simulink model "AVION_LONGITUDINAL"  (Simulink 8.2)
settings: Solver=ode45  StartTime=0.0  StopTime=100  RelTol=1e-8
values from neighbouring files (symbols this model uses):
  ACinertia_yy = 8000.0    (= 8000)    [iniAVION_LONGITUDINAL.m]
  ACmass = 90000.0    (= 90000)    [iniAVION_LONGITUDINAL.m]
  ae = Ue(2)    [iniAVION_LONGITUDINAL.m]
  cbar = 5.0    (= 5)    [iniAVION_LONGITUDINAL.m]
  CD0 = 0.018    [iniAVION_LONGITUDINAL.m]
  CD1 = 0.009    [iniAVION_LONGITUDINAL.m]
  CD2 = 0.040    (= 0.04)    [iniAVION_LONGITUDINAL.m]
  CL0 = 0.20    (= 0.2)    [iniAVION_LONGITUDINAL.m]
  CLalfa = 0.20    (= 0.2)    [iniAVION_LONGITUDINAL.m]
  CM0 = 0.050    (= 0.05)    [iniAVION_LONGITUDINAL.m]
  CMalfa = -0.001    [iniAVION_LONGITUDINAL.m]
  CMdelta = -0.016    [iniAVION_LONGITUDINAL.m]
  CMq = -0.300    (= -0.3)    [iniAVION_LONGITUDINAL.m]
  d2r_cst = pi/180.0    (= 0.0174532925199)    [iniAVION_LONGITUDINAL.m]
  deltae = Ue(1)    [iniAVION_LONGITUDINAL.m]
  etat_ini = etat_equil    [iniAVION_LONGITUDINAL.m]
  FT80 = thrust_max    (= 108000)    [iniAVION_LONGITUDINAL.m]
  FT_V = -200.0    (= -200)    [iniAVION_LONGITUDINAL.m]
  g_cst = 9.78    [iniAVION_LONGITUDINAL.m]
  pos_ini = [h_ini, pN_ini]    [iniAVION_LONGITUDINAL.m]
  r2d_cst = 1.0/d2r_cst    (= 57.2957795131)    [iniAVION_LONGITUDINAL.m]
  rho = 1.225    [iniAVION_LONGITUDINAL.m]
  Sref = 200.0    (= 200)    [iniAVION_LONGITUDINAL.m]
  xt = -0.3    [iniAVION_LONGITUDINAL.m]
undefined symbols (not defined in the file or in its folder): A, B, C, D, Ye
settings Model: Creator=delafontaine  LastModifiedBy=Ouss
settings DataIOCC: SignalLoggingName=sigsOut
settings OptimizationCC: BooleanDataType=off
settings DebuggingCC: SaveWithParameterizedLinksMsg=none  SignalResolutionControl=TryResolveAllWithWarning  SolverPrmCheckMsg=none  MultiTaskDSMMsg=warning  MultiTaskCondExecSysMsg=none  FcnCallInpInsideContextMsg=EnableAllAsWarning  FrameProcessingCompatibilityMsg=error
settings HardwareCC: TargetUnknown=on
settings GRTTargetCC: CodeReplacementLibrary=None  CPPClassGenCompliant=on

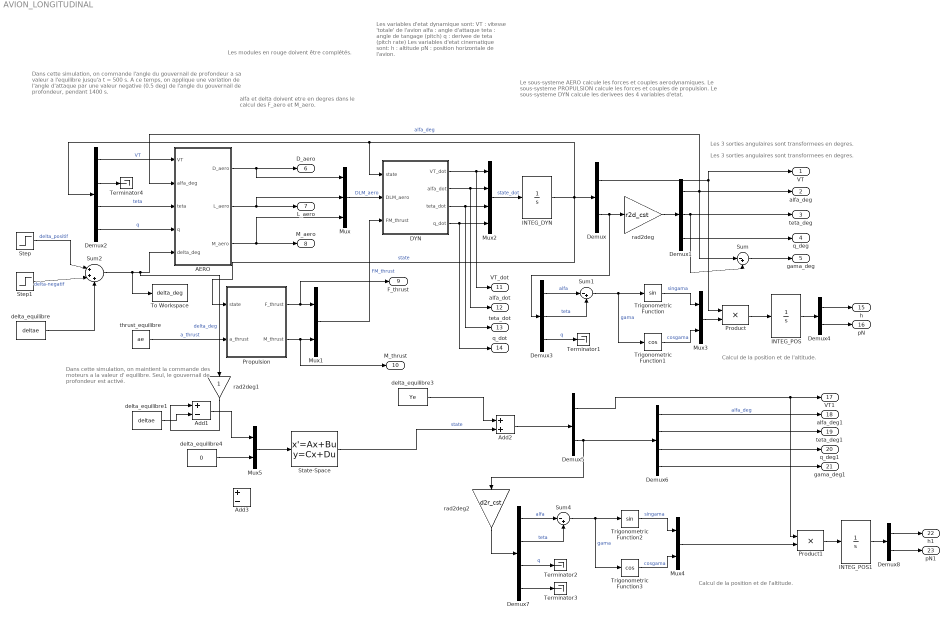
== system AVION_LONGITUDINAL ==
  note: Dans cette simulation, on commande l'angle du gouvernail
      | de profondeur a sa valeur a l'equilibre jusqu'a t = 500 s. A ce
      | temps, on applique une variation de l'angle d'attaque
      | par une valeur negative (0.5 deg) de l'angle du gouvernail
      | de profondeur, pendant 1400 s.
  note: alfa et delta doivent etre en degres
      | dans le calcul des F_aero et M_aero.
  note: Les variables d'etat dynamique sont:
      |
      | VT   : vitesse 'totale' de l'avion
      | alfa : angle d'attaque
      | teta : angle de tangage (pitch)
      | q    : derivee de teta (pitch rate)
      |
      | Les variables d'etat cinematique sont:
      |
      | h    : altitude
      | pN   : position horizontale de l'avion.
  note: Les 3 sorties angulaires sont transformees en degres.
  note: Calcul de la position et de l'altitude.
  note: Le sous-systeme AERO calcule les forces et couples
      | aerodynamiques. Le sous-systeme PROPULSION calcule
      | les forces et couples de propulsion. Le sous-systeme
      | DYN calcule les derivees des 4 variables d'etat.
  note: Dans cette simulation, on maintient la
      | commande des moteurs a la valeur d' equilibre.
      | Seul, le gouvernail de profondeur est activé.
  note: Les modules en rouge doivent être complétés.
  note: Les 3 sorties angulaires sont transformees en degres.
  note: Calcul de la position et de l'altitude.
  AERO : Subsystem
  Add1 : Sum  Inputs=+-
  Add2 : Sum
  Add3 : Sum  Inputs=+-
  DYN : Subsystem
  Demux : Demux  Outputs=[1,3]
  Demux1 : Demux  Outputs=3
  Demux2 : Demux
  Demux3 : Demux  Outputs=3
  Demux4 : Demux  Outputs=2
  Demux5 : Demux  Outputs=[1,4]
  Demux6 : Demux
  Demux7 : Demux
  Demux8 : Demux  Outputs=2
  INTEG_DYN : Integrator  InitialCondition=etat_ini
  INTEG_POS : Integrator  InitialCondition=pos_ini
  INTEG_POS1 : Integrator  InitialCondition=pos_ini
  Mux : Mux  Inputs=3
  Mux{1,3..5} (4 alike) : Mux  Inputs=2
  Mux2 : Mux
  Product : Product  Inputs=**  SaturateOnIntegerOverflow=on  InputSameDT=on  OutDataTypeStr=Inherit: Same as first input
  Product1 : Product  Inputs=**  SaturateOnIntegerOverflow=on  InputSameDT=on  OutDataTypeStr=Inherit: Same as first input
  Propulsion : Subsystem
  State-Space : StateSpace  A=A  B=B  C=C  D=D  X0=0  ContinuousStateAttributes='avionnn'
  Step : Step  Time=1900  After=0.5  SampleTime=0
  Step1 : Step  Time=500  After=-0.5  SampleTime=0
  Sum : Sum  Inputs=|-+  SaturateOnIntegerOverflow=on  InputSameDT=on  OutDataTypeStr=Inherit: Same as first input
  Sum1 : Sum  Inputs=|-+  SaturateOnIntegerOverflow=on  InputSameDT=on  OutDataTypeStr=Inherit: Same as first input
  Sum2 : Sum  Inputs=|+++  SaturateOnIntegerOverflow=on  InputSameDT=on  OutDataTypeStr=Inherit: Same as first input
  Sum4 : Sum  Inputs=|-+  SaturateOnIntegerOverflow=on  InputSameDT=on  OutDataTypeStr=Inherit: Same as first input
  Terminator{1..4} (4 alike) : Terminator
  To Workspace : ToWorkspace  VariableName=delta_deg  SampleTime=-1
  Trigonometric Function : Trigonometry
  Trigonometric Function1 : Trigonometry  Operator=cos
  Trigonometric Function2 : Trigonometry
  Trigonometric Function3 : Trigonometry  Operator=cos
  delta_equilibre : Constant  Value=deltae
  delta_equilibre1 : Constant  Value=deltae
  delta_equilibre3 : Constant  Value=Ye
  delta_equilibre4 : Constant  Value=0
  rad2deg : Gain  Gain=r2d_cst  SaturateOnIntegerOverflow=on  OutDataTypeStr=Inherit: Same as input  ParamDataTypeStr=Inherit: Same as input
  rad2deg1 : Gain  SaturateOnIntegerOverflow=on  OutDataTypeStr=Inherit: Same as input  ParamDataTypeStr=Inherit: Same as input
  rad2deg2 : Gain  Gain=d2r_cst  SaturateOnIntegerOverflow=on  OutDataTypeStr=Inherit: Same as input  ParamDataTypeStr=Inherit: Same as input
  thrust_equilibre : Constant  Value=ae
  VT : Outport
  alfa_deg : Outport  Port=2
  teta_deg : Outport  Port=3
  q_deg : Outport  Port=4
  gama_deg : Outport  Port=5
  D_aero : Outport  Port=6
  L_aero : Outport  Port=7
  M_aero : Outport  Port=8
  F_thrust : Outport  Port=9
  M_thrust : Outport  Port=10
  VT_dot : Outport  Port=11
  alfa_dot : Outport  Port=12
  teta_dot : Outport  Port=13
  q_dot : Outport  Port=14
  h : Outport  Port=15
  pN : Outport  Port=16
  VT1 : Outport  Port=17
  alfa_deg1 : Outport  Port=18
  teta_deg1 : Outport  Port=19
  q_deg1 : Outport  Port=20
  gama_deg1 : Outport  Port=21
  h1 : Outport  Port=22
  pN1 : Outport  Port=23
  wires:
  AERO/1(D_aero) -> D_aero/1, Mux/1
  AERO/2(L_aero) -> L_aero/1, Mux/2
  AERO/3(M_aero) -> M_aero/1, Mux/3
  Mux/1 -> DYN/2(DLM_aero)  "DLM_aero"
  Propulsion/1(F_thrust) -> Mux1/1, F_thrust/1
  Propulsion/2(M_thrust) -> Mux1/2, M_thrust/1
  Mux1/1 -> DYN/3(FM_thrust)  "FM_thrust"
  thrust_equilibre/1 -> Propulsion/2(a_thrust)  "a_thrust"
  DYN/1(VT_dot) -> Mux2/1, VT_dot/1
  DYN/2(alfa_dot) -> Mux2/2, alfa_dot/1
  DYN/3(teta_dot) -> Mux2/3, teta_dot/1
  DYN/4(q_dot) -> Mux2/4, q_dot/1
  Mux2/1 -> INTEG_DYN/1  "state_dot"
  INTEG_DYN/1 -> Demux/1, Demux2/1, DYN/1(state), Propulsion/1(state)  "state"
  Demux/2 -> rad2deg/1, Demux3/1
  Demux/1 -> Product/1, VT/1
  rad2deg/1 -> Demux1/1
  Demux1/1 -> AERO/2(alfa_deg), alfa_deg/1, Sum/1  "alfa_deg"
  Demux1/2 -> teta_deg/1, Sum/2
  Demux1/3 -> q_deg/1
  Sum/1 -> gama_deg/1
  Demux2/1 -> AERO/1(VT)  "VT"
  Demux2/3 -> AERO/3(teta)  "teta"
  Demux2/4 -> AERO/4(q)  "q"
  Sum1/1 -> Trigonometric Function/1, Trigonometric Function1/1  "gama"
  Trigonometric Function/1 -> Mux3/1  "singama"
  Trigonometric Function1/1 -> Mux3/2  "cosgama"
  INTEG_POS/1 -> Demux4/1
  Demux4/1 -> h/1
  Demux4/2 -> pN/1
  Demux3/3 -> Terminator1/1  "q"
  Demux3/1 -> Sum1/1  "alfa"
  Demux3/2 -> Sum1/2  "teta"
  delta_equilibre/1 -> Sum2/3
  Sum2/1 -> rad2deg1/1, AERO/5(delta_deg), To Workspace/1  "delta_deg"
  Step/1 -> Sum2/1  "delta_positif"
  Step1/1 -> Sum2/2  "delta-negatif"
  Mux3/1 -> Product/2
  Product/1 -> INTEG_POS/1
  Sum4/1 -> Trigonometric Function3/1, Trigonometric Function2/1  "gama"
  Trigonometric Function2/1 -> Mux4/1  "singama"
  Trigonometric Function3/1 -> Mux4/2  "cosgama"
  INTEG_POS1/1 -> Demux8/1
  Demux8/1 -> h1/1
  Demux8/2 -> pN1/1
  Demux7/3 -> Terminator2/1  "q"
  Demux7/1 -> Sum4/1  "alfa"
  Demux7/2 -> Sum4/2  "teta"
  Demux7/4 -> Terminator3/1
  Mux5/1 -> State-Space/1
  delta_equilibre1/1 -> Add1/2
  Add1/1 -> Mux5/1
  Demux6/1 -> alfa_deg1/1  "alfa_deg"
  Demux5/1 -> Product1/1, VT1/1
  Demux6/2 -> teta_deg1/1
  Demux6/3 -> q_deg1/1
  Demux6/4 -> gama_deg1/1
  Product1/1 -> INTEG_POS1/1
  rad2deg1/1 -> Add1/1
  Mux4/1 -> Product1/2
  rad2deg2/1 -> Demux7/1
  Add2/1 -> Demux5/1
  State-Space/1 -> Add2/2  "state"
  delta_equilibre3/1 -> Add2/1
  delta_equilibre4/1 -> Mux5/2
  Demux5/2 -> Demux6/1, rad2deg2/1
  Demux2/2 -> Terminator4/1

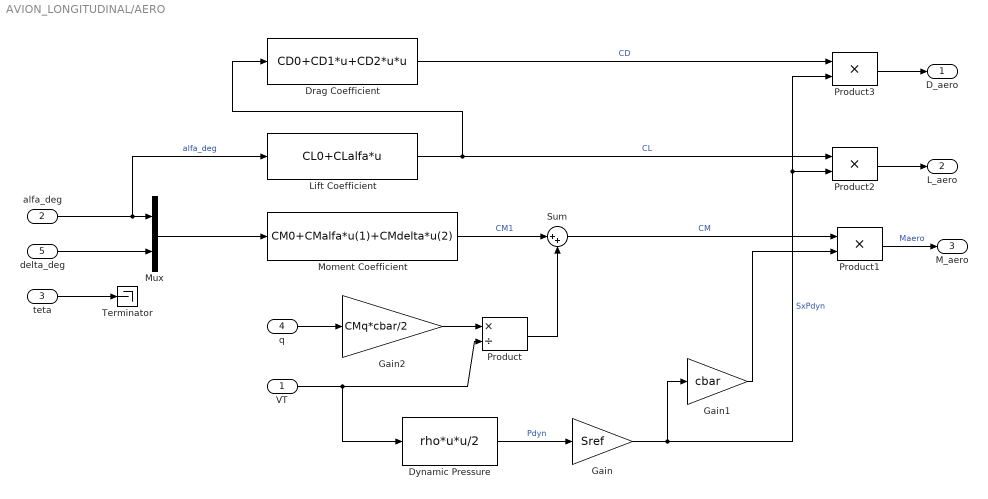
== system AVION_LONGITUDINAL/AERO ==
  VT : Inport
  alfa_deg : Inport  Port=2
  teta : Inport  Port=3
  q : Inport  Port=4
  delta_deg : Inport  Port=5
  Drag Coefficient : Fcn  Expr=CD0+CD1*u+CD2*u*u
  Dynamic Pressure : Fcn  Expr=rho*u*u/2
  Gain : Gain  Gain=Sref  SaturateOnIntegerOverflow=on  OutDataTypeStr=Inherit: Same as input  ParamDataTypeStr=Inherit: Same as input
  Gain1 : Gain  Gain=cbar  SaturateOnIntegerOverflow=on  OutDataTypeStr=Inherit: Same as input  ParamDataTypeStr=Inherit: Same as input
  Gain2 : Gain  Gain=CMq*cbar/2  SaturateOnIntegerOverflow=on  OutDataTypeStr=Inherit: Same as input  ParamDataTypeStr=Inherit: Same as input
  Lift Coefficient : Fcn  Expr=CL0+CLalfa*u
  Moment Coefficient : Fcn  Expr=CM0+CMalfa*u(1)+CMdelta*u(2)
  Mux : Mux  Inputs=2
  Product : Product  Inputs=*/  SaturateOnIntegerOverflow=on  InputSameDT=on  OutDataTypeStr=Inherit: Same as first input
  Product1 : Product  Inputs=**  SaturateOnIntegerOverflow=on  InputSameDT=on  OutDataTypeStr=Inherit: Same as first input
  Product2 : Product  Inputs=**  SaturateOnIntegerOverflow=on  InputSameDT=on  OutDataTypeStr=Inherit: Same as first input
  Product3 : Product  Inputs=**  SaturateOnIntegerOverflow=on  InputSameDT=on  OutDataTypeStr=Inherit: Same as first input
  Sum : Sum  Inputs=|++  SaturateOnIntegerOverflow=on  InputSameDT=on  OutDataTypeStr=Inherit: Same as first input
  Terminator : Terminator
  D_aero : Outport
  L_aero : Outport  Port=2
  M_aero : Outport  Port=3
  wires:
  Dynamic Pressure/1 -> Gain/1  "Pdyn"
  q/1 -> Gain2/1
  Gain2/1 -> Product/1
  VT/1 -> Product/2, Dynamic Pressure/1
  Product/1 -> Sum/2
  Moment Coefficient/1 -> Sum/1  "CM1"
  Sum/1 -> Product1/1  "CM"
  alfa_deg/1 -> Lift Coefficient/1, Mux/1  "alfa_deg"
  delta_deg/1 -> Mux/2
  Mux/1 -> Moment Coefficient/1
  Gain1/1 -> Product1/2
  Product1/1 -> M_aero/1  "Maero"
  Lift Coefficient/1 -> Drag Coefficient/1, Product2/1  "CL"
  Drag Coefficient/1 -> Product3/1  "CD"
  Product3/1 -> D_aero/1
  Product2/1 -> L_aero/1
  teta/1 -> Terminator/1
  Gain/1 -> Product2/2, Product3/2, Gain1/1  "SxPdyn"

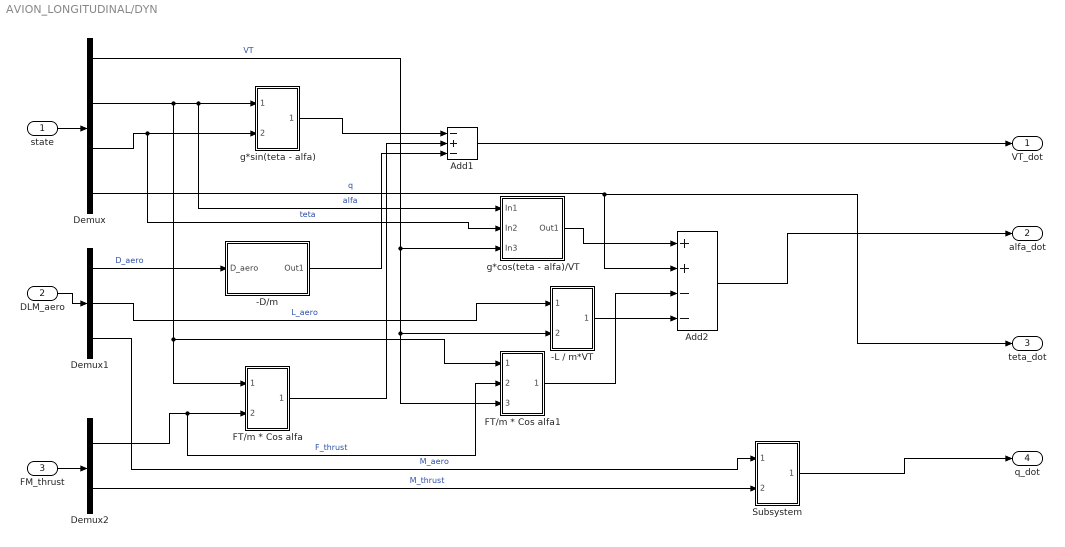
== system AVION_LONGITUDINAL/DYN ==
  state : Inport
  DLM_aero : Inport  Port=2
  FM_thrust : Inport  Port=3
  -D/m : Subsystem
  -L / m*VT : Subsystem
  Add1 : Sum  Inputs=-+-
  Add2 : Sum  Inputs=++--
  Demux : Demux
  Demux1 : Demux  Outputs=3
  Demux2 : Demux  Outputs=2
  FT/m * Cos alfa : Subsystem
  FT/m * Cos alfa1 : Subsystem
  Subsystem : Subsystem
  g*cos(teta - alfa)/VT : Subsystem
  g*sin(teta - alfa) : Subsystem
  VT_dot : Outport
  alfa_dot : Outport  Port=2
  teta_dot : Outport  Port=3
  q_dot : Outport  Port=4
  wires:
  state/1 -> Demux/1
  Demux/1 -> -L / m*VT/2(In2), FT/m * Cos alfa1/3(In3), g*cos(teta - alfa)/VT/3(In3)  "VT"
  DLM_aero/1 -> Demux1/1
  FM_thrust/1 -> Demux2/1
  Demux/2 -> FT/m * Cos alfa1/1(In1), FT/m * Cos alfa/1(In1), g*cos(teta - alfa)/VT/1(In1), g*sin(teta - alfa)/1(In1)  "alfa"
  Demux/4 -> teta_dot/1, Add2/2  "q"
  Demux1/2 -> -L / m*VT/1(In1)  "L_aero"
  Add1/1 -> VT_dot/1
  Demux2/1 -> FT/m * Cos alfa1/2(In2), FT/m * Cos alfa/2(In2)  "F_thrust"
  FT/m * Cos alfa/1(Out1) -> Add1/2
  Demux1/1 -> -D/m/1("D_aero ")  "D_aero"
  -D/m/1(Out1) -> Add1/3
  Demux/3 -> g*cos(teta - alfa)/VT/2(In2), g*sin(teta - alfa)/2(In2)  "teta"
  g*sin(teta - alfa)/1(Out1) -> Add1/1
  g*cos(teta - alfa)/VT/1(Out1) -> Add2/1
  FT/m * Cos alfa1/1(Out1) -> Add2/3
  -L / m*VT/1(Out1) -> Add2/4
  Add2/1 -> alfa_dot/1
  Demux1/3 -> Subsystem/1(In1)  "M_aero"
  Demux2/2 -> Subsystem/2(In2)  "M_thrust"
  Subsystem/1(Out1) -> q_dot/1

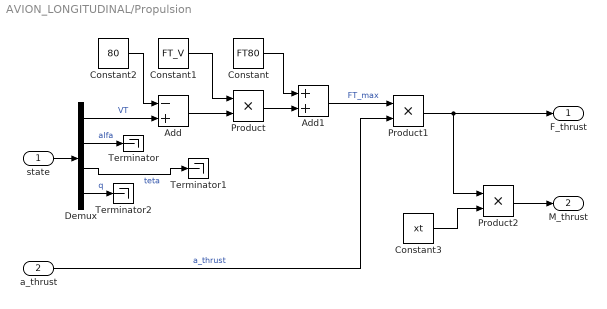
== system AVION_LONGITUDINAL/Propulsion ==
  state : Inport
  a_thrust : Inport  Port=2
  Add : Sum  Inputs=-+
  Add1 : Sum
  Constant : Constant  Value=FT80
  Constant1 : Constant  Value=FT_V
  Constant2 : Constant  Value=80
  Constant3 : Constant  Value=xt
  Demux : Demux
  Product : Product
  Product1 : Product
  Product2 : Product
  Terminator : Terminator
  Terminator1 : Terminator
  Terminator2 : Terminator
  F_thrust : Outport
  M_thrust : Outport  Port=2
  wires:
  state/1 -> Demux/1
  Demux/1 -> Add/2  "VT"
  Demux/3 -> Terminator1/1  "teta"
  Demux/4 -> Terminator2/1  "q"
  a_thrust/1 -> Product1/2  "a_thrust"
  Constant2/1 -> Add/1
  Constant1/1 -> Product/1
  Add/1 -> Product/2
  Product/1 -> Add1/2
  Constant/1 -> Add1/1
  Add1/1 -> Product1/1  "FT_max"
  Product1/1 -> Product2/1, F_thrust/1
  Demux/2 -> Terminator/1  "alfa"
  Constant3/1 -> Product2/2
  Product2/1 -> M_thrust/1

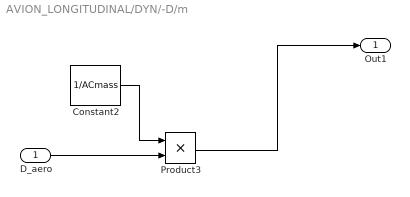
== system AVION_LONGITUDINAL/DYN/-D/m ==
  "D_aero " : Inport
  Constant2 : Constant  Value=1/ACmass
  Product3 : Product
  Out1 : Outport
  wires:
  Product3/1 -> Out1/1
  Constant2/1 -> Product3/1
  "D_aero "/1 -> Product3/2

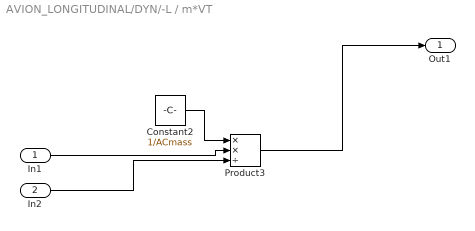
== system AVION_LONGITUDINAL/DYN/-L / m*VT ==
  In1 : Inport
  In2 : Inport  Port=2
  Constant2 : Constant  Value=1/ACmass
  Product3 : Product  Inputs=**/
  Out1 : Outport
  wires:
  In1/1 -> Product3/2
  Constant2/1 -> Product3/1
  Product3/1 -> Out1/1
  In2/1 -> Product3/3

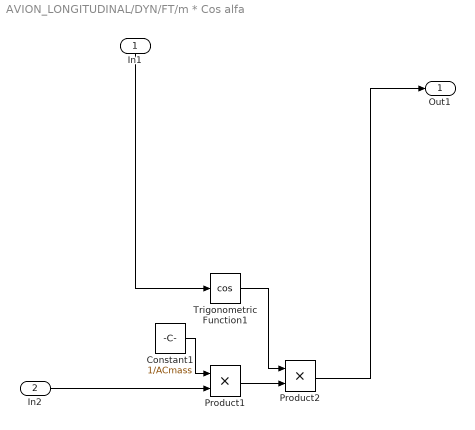
== system AVION_LONGITUDINAL/DYN/FT/m * Cos alfa ==
  In1 : Inport
  In2 : Inport  Port=2
  Constant1 : Constant  Value=1/ACmass
  Product1 : Product
  Product2 : Product
  Trigonometric Function1 : Trigonometry  Operator=cos
  Out1 : Outport
  wires:
  Product1/1 -> Product2/2
  Constant1/1 -> Product1/1
  In1/1 -> Trigonometric Function1/1
  Trigonometric Function1/1 -> Product2/1
  Product2/1 -> Out1/1
  In2/1 -> Product1/2

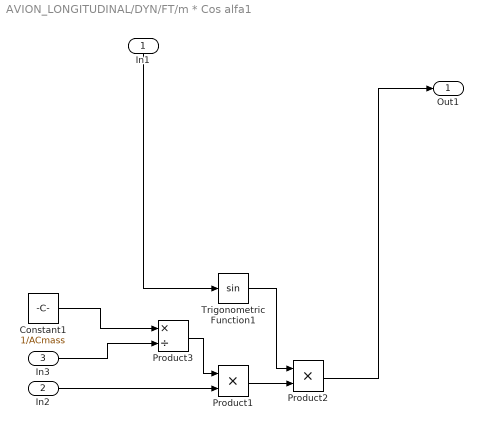
== system AVION_LONGITUDINAL/DYN/FT/m * Cos alfa1 ==
  In1 : Inport
  In2 : Inport  Port=2
  In3 : Inport  Port=3
  Constant1 : Constant  Value=1/ACmass
  Product1 : Product
  Product2 : Product
  Product3 : Product  Inputs=*/
  Trigonometric Function1 : Trigonometry
  Out1 : Outport
  wires:
  In2/1 -> Product1/2
  Product2/1 -> Out1/1
  Trigonometric Function1/1 -> Product2/1
  In1/1 -> Trigonometric Function1/1
  Product1/1 -> Product2/2
  Product3/1 -> Product1/1
  Constant1/1 -> Product3/1
  In3/1 -> Product3/2

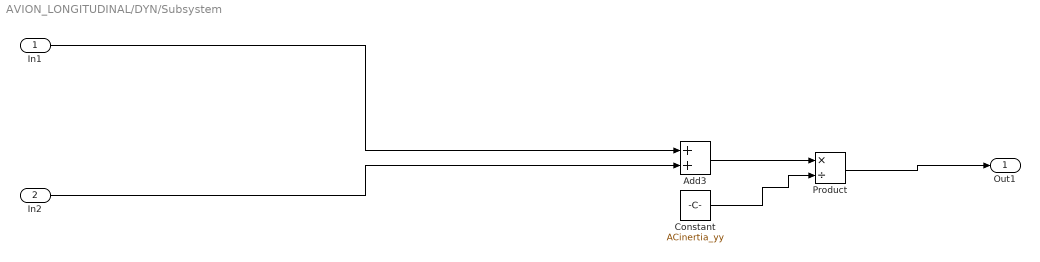
== system AVION_LONGITUDINAL/DYN/Subsystem ==
  In1 : Inport
  In2 : Inport  Port=2
  Add3 : Sum
  Constant : Constant  Value=ACinertia_yy
  Product : Product  Inputs=*/
  Out1 : Outport
  wires:
  Product/1 -> Out1/1
  Add3/1 -> Product/1
  In2/1 -> Add3/2
  In1/1 -> Add3/1
  Constant/1 -> Product/2

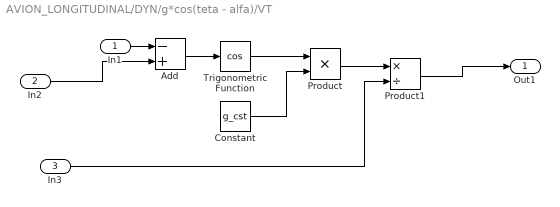
== system AVION_LONGITUDINAL/DYN/g*cos(teta - alfa)/VT ==
  In1 : Inport
  In2 : Inport  Port=2
  In3 : Inport  Port=3
  Add : Sum  Inputs=-+
  Constant : Constant  Value=g_cst
  Product : Product
  Product1 : Product  Inputs=*/
  Trigonometric Function : Trigonometry  Operator=cos
  Out1 : Outport
  wires:
  Add/1 -> Trigonometric Function/1
  In2/1 -> Add/2
  In1/1 -> Add/1
  Constant/1 -> Product/2
  Trigonometric Function/1 -> Product/1
  Product1/1 -> Out1/1
  Product/1 -> Product1/1
  In3/1 -> Product1/2

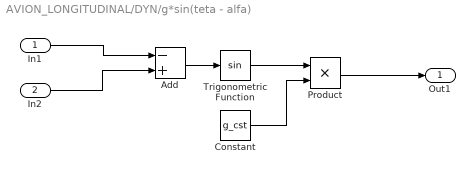
== system AVION_LONGITUDINAL/DYN/g*sin(teta - alfa) ==
  In1 : Inport
  In2 : Inport  Port=2
  Add : Sum  Inputs=-+
  Constant : Constant  Value=g_cst
  Product : Product
  Trigonometric Function : Trigonometry
  Out1 : Outport
  wires:
  Product/1 -> Out1/1
  Trigonometric Function/1 -> Product/1
  Constant/1 -> Product/2
  In1/1 -> Add/1
  In2/1 -> Add/2
  Add/1 -> Trigonometric Function/1
